simulink model "AEB"  (R2018b)
settings: Solver=FixedStepAuto  StartTime=0.0  StopTime=100  FixedStep=0.001  RelTol=1e-3  EnableMultiTasking=on
libraries: embdlinuxlib x2, raspberrypilib x2
settings Model: SimulationMode=external  Creator=李东峻  LastModifiedBy=李东峻
settings SolverCC: PositivePriorityOrder=on
settings OptimizationCC: EnhancedBackFolding=on  PassReuseOutputArgsAs=Individual arguments  MaxStackSize=64  OptimizeBlockOrder=speed  DifferentSizesBufferReuse=on  OptimizationCustomize=off
settings DebuggingCC: ParameterTunabilityLossMsg=error
settings HardwareCC: ProdBitPerPointer=32  ProdBitPerSizeT=32  ProdBitPerPtrDiffT=32  ProdLargestAtomicInteger=Long  ProdLargestAtomicFloat=Double  ProdWordSize=32  ProdHWDeviceType=ARM Compatible->ARM Cortex
settings SFSimCC: MATLABDynamicMemAlloc=off
settings RTWCC: SystemTargetFile=ert.tlc  HardwareBoard=Raspberry Pi  TLCOptions="-aInlineSetEventsForThisBaseRateFcn=TLC_FALSE -aSuppressMultiTaskScheduler=TLC_FALSE  -aRateBasedStepFcn=0"  TemplateMakefile=ert_default_tmf  GenerateReport=on  Toolchain=GNU GCC Raspberry Pi  BuildConfiguration=Faster Runs  IncludeHyperlinkInReport=on  LaunchReport=on  GenerateTraceInfo=on  GenerateTraceReport=on  GenerateTraceReportSl=on  GenerateTraceReportSf=on  GenerateTraceReportEml=on
settings CodeAppCC: ForceParamTrailComments=on  IgnoreCustomStorageClasses=off  OperatorAnnotations=on  SimulinkDataObjDesc=on  SFDataObjDesc=on  InsertBlockDesc=on
settings ERTTargetCC: SupportContinuousTime=on  SupportVariableSizeSignals=on  ExtMode=on  ExtModeMexArgs='192.168.43.49' 0 17725

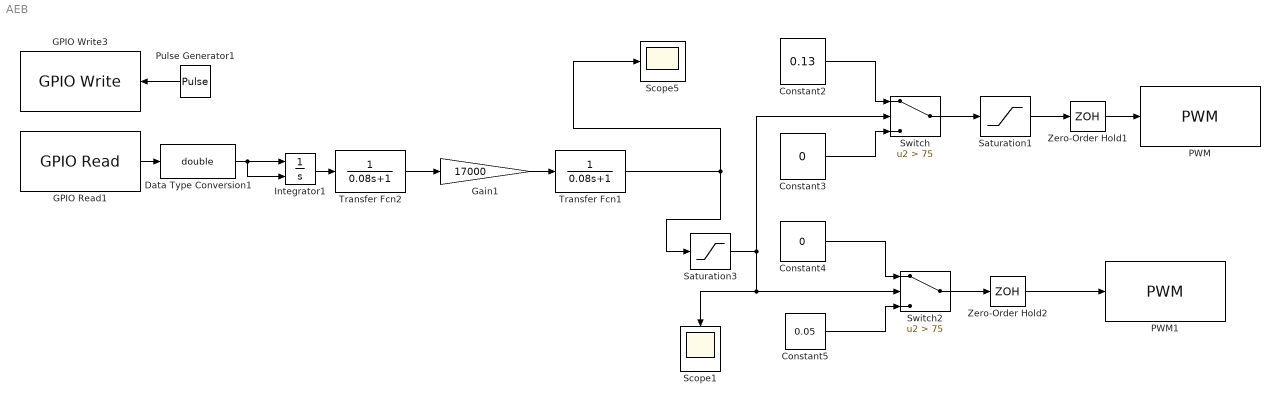
== system AEB ==
  Constant2 : Constant  Value=0.13
  Constant3 : Constant  Value=0
  Constant4 : Constant  Value=0
  Constant5 : Constant  Value=0.05
  Data Type Conversion1 : DataTypeConversion  OutDataTypeStr=double
  GPIO Read1 : embdlinuxlib/GPIO Read  board=Pi 3 Model B+  gpio=24  internalResistor=Off  sampleTime=inf  direction=Input  blockPlatform=Raspberry Pi
      settings: SourceProductName=Simulink Support Package for Raspberry Pi Hardware  SourceProductBaseCode=RASPPI
  GPIO Write3 : embdlinuxlib/GPIO Write  board=Pi 3 Model B+  gpio=23  direction=Output  blockPlatform=Raspberry Pi
      settings: SourceProductName=Simulink Support Package for Raspberry Pi Hardware  SourceProductBaseCode=RASPPI
  Gain1 : Gain  Gain=17000
  Integrator1 : Integrator  ExternalReset=rising
  PWM : raspberrypilib/PWM  board=Pi 3 Model B  Pin_=17  Frequency=800  blockPlatform=Raspberry Pi
      settings: SourceProductName=Simulink Support Package for Raspberry Pi Hardware  SourceProductBaseCode=RASPPI
  PWM1 : raspberrypilib/PWM  board=Pi 3 Model B  Pin_=27  Frequency=800  blockPlatform=Raspberry Pi
      settings: SourceProductName=Simulink Support Package for Raspberry Pi Hardware  SourceProductBaseCode=RASPPI
  Pulse Generator1 : DiscretePulseGenerator  PulseType=Time based  Period=0.1  PulseWidth=50
  Saturation1 : Saturate  UpperLimit=0.2  LowerLimit=0
  Saturation3 : Saturate  UpperLimit=100  LowerLimit=0
  Scope1 : Scope
  Scope5 : Scope
  Switch : Switch  Criteria=u2 > Threshold  Threshold=75
  Switch2 : Switch  Criteria=u2 > Threshold  Threshold=75
  Transfer Fcn1 : TransferFcn  Denominator=[0.08 1]
  Transfer Fcn2 : TransferFcn  Denominator=[0.08 1]
  Zero-Order Hold1 : ZeroOrderHold  SampleTime=0.5
  Zero-Order Hold2 : ZeroOrderHold  SampleTime=0.5
  wires:
  Saturation1/1 -> Zero-Order Hold1/1
  Saturation3/1 -> Scope1/1, Switch2/2, Switch/2
  Switch2/1 -> Zero-Order Hold2/1
  Data Type Conversion1/1 -> Integrator1/2, Integrator1/1
  Gain1/1 -> Transfer Fcn1/1
  Integrator1/1 -> Transfer Fcn2/1
  Pulse Generator1/1 -> GPIO Write3/1
  GPIO Read1/1 -> Data Type Conversion1/1
  Transfer Fcn2/1 -> Gain1/1
  Zero-Order Hold1/1 -> PWM/1
  Zero-Order Hold2/1 -> PWM1/1
  Constant2/1 -> Switch/1
  Constant3/1 -> Switch/3
  Switch/1 -> Saturation1/1
  Constant4/1 -> Switch2/1
  Constant5/1 -> Switch2/3
  Transfer Fcn1/1 -> Saturation3/1, Scope5/1
